simulink model "actualproject"  (R2020b)
settings: Solver=VariableStepAuto  StartTime=0.0  StopTime=25  RelTol=1e-3
libraries: simulink x2
settings Model: Creator=mori  LastModifiedBy=mori

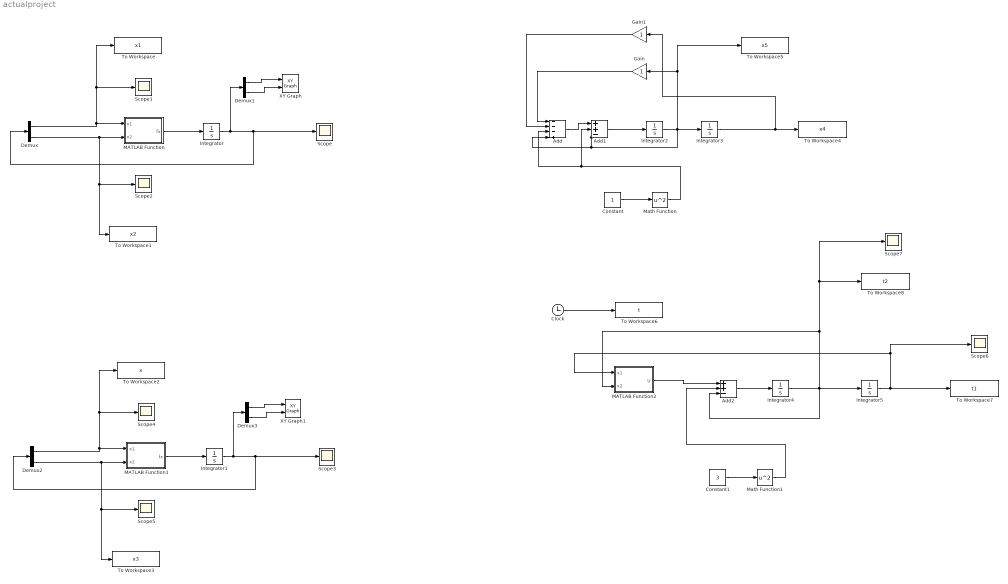
== system actualproject ==
  Add : Sum  Inputs=---+
  Add1 : Sum  Inputs=++-
  Add2 : Sum  Inputs=++-
  Clock : Clock
  Constant : Constant
  Constant1 : Constant  Value=3
  Demux{,1..3} (4 alike) : Demux  Outputs=2
  Gain : Gain
  Gain1 : Gain
  Integrator{,1..5} (6 alike) : Integrator  InitialCondition=[0.75;0]
  MATLAB Function : MATLAB Function  TreatAsAtomicUnit=on
  MATLAB Function1 : MATLAB Function  TreatAsAtomicUnit=on
  MATLAB Function2 : MATLAB Function  TreatAsAtomicUnit=on
  Math Function : Math  Operator=square  OutputSignalType=complex  SaturateOnIntegerOverflow=on
  Math Function1 : Math  Operator=square  OutputSignalType=complex  SaturateOnIntegerOverflow=on
  Scope{,1..7} (8 alike) : Scope
  To Workspace : ToWorkspace  VariableName=x1  SaveFormat=Timeseries  SampleTime=-1
  To Workspace1 : ToWorkspace  VariableName=x2  SaveFormat=Timeseries  SampleTime=-1
  To Workspace2 : ToWorkspace  VariableName=x  SaveFormat=Timeseries  SampleTime=-1
  To Workspace3 : ToWorkspace  VariableName=x3  SaveFormat=Timeseries  SampleTime=-1
  To Workspace4 : ToWorkspace  VariableName=x4  SaveFormat=Timeseries  SampleTime=-1
  To Workspace5 : ToWorkspace  VariableName=x5  SaveFormat=Timeseries  SampleTime=-1
  To Workspace6 : ToWorkspace  VariableName=t  SaveFormat=Timeseries  SampleTime=-1
  To Workspace7 : ToWorkspace  VariableName=t1  SaveFormat=Timeseries  SampleTime=-1
  To Workspace8 : ToWorkspace  VariableName=t2  SaveFormat=Timeseries  SampleTime=-1
  XY Graph : simulink/Sinks/XY Graph  xmin=-1  xmax=1  ymin=-1  ymax=1  st=-1
  XY Graph1 : simulink/Sinks/XY Graph  xmin=-1  xmax=1  ymin=-1  ymax=1  st=-1
  wires:
  MATLAB Function/1(fx) -> Integrator/1
  Demux/1 -> To Workspace/1, Scope1/1, MATLAB Function/1(x1)
  Integrator/1 -> Demux1/1, Demux/1, Scope/1
  Demux/2 -> To Workspace1/1, Scope2/1, MATLAB Function/2(x2)
  Demux1/1 -> XY Graph/1
  Demux1/2 -> XY Graph/2
  Demux3/1 -> XY Graph1/1
  Demux3/2 -> XY Graph1/2
  Integrator1/1 -> Demux3/1, Demux2/1, Scope3/1
  Demux2/1 -> To Workspace2/1, Scope4/1, MATLAB Function1/1(x1)
  Demux2/2 -> To Workspace3/1, Scope5/1, MATLAB Function1/2(x2)
  MATLAB Function1/1(fx) -> Integrator1/1
  Constant/1 -> Math Function/1
  Gain/1 -> Add/1
  Gain1/1 -> Add/2
  Integrator2/1 -> Add1/3, Add/4, To Workspace5/1, Gain/1, Integrator3/1
  Add/1 -> Add1/1
  Math Function/1 -> Add1/2, Add/3
  Add1/1 -> Integrator2/1
  Integrator3/1 -> Gain1/1, To Workspace4/1
  MATLAB Function2/1(U) -> Add2/1
  Constant1/1 -> Math Function1/1
  Math Function1/1 -> Add2/2
  Add2/1 -> Integrator4/1
  Integrator4/1 -> Add2/3, Scope7/1, To Workspace8/1, MATLAB Function2/2(x2), Integrator5/1
  Integrator5/1 -> To Workspace7/1, Scope6/1, MATLAB Function2/1(x1)
  Clock/1 -> To Workspace6/1

== matlab function actualproject/MATLAB Function ==
  data: x1 input; fx output; x2 input
function fx = fcn(x1,x2)
A=[0 1;-1 -1];
X=[x1;x2];

fx=A*X

== matlab function actualproject/MATLAB Function2 ==
  data: x1 input; U output; x2 input
function U = fcn(x1,x2)
A=[0 1;-1 -1];
X=[x1;x2];

U=A*X

== matlab function actualproject/MATLAB Function1 ==
  data: x1 input; fx output; x2 input
function fx=fcn(x1,x2)
A = [0 1;-1 -1];
X =[x1;x2];
B =[0;-sin(x1)+sin(x2)];
fx = (A*X)+B;
